simulink model "Project5_openloop"  (R2014b)
settings: Solver=ode5  StartTime=0.0  StopTime=10  FixedStep=0.01  RelTol=1e-3
settings Model: Creator=axk7578  LastModifiedBy=axk7578

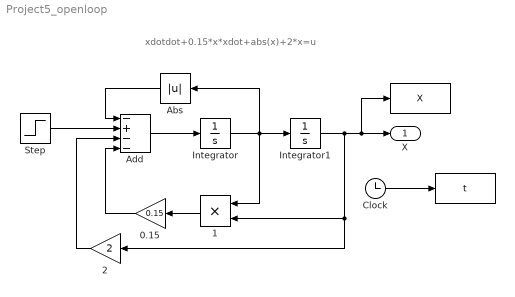
== system Project5_openloop ==
  note: xdotdot+0.15*x*xdot+abs(x)+2*x=u
  " " : ToWorkspace  VariableName=t  SampleTime=-1
  " " : ToWorkspace  VariableName=X  SampleTime=-1
  " 1" : Product
  0.15 : Gain  Gain=0.15
  2 : Gain  Gain=2
  Abs : Abs
  Add : Sum  Inputs=-+--
  Clock : Clock
  Integrator : Integrator
  Integrator1 : Integrator
  Step : Step  Time=0  SampleTime=0
  X : Outport
  wires:
  Clock/1 -> " "/1
  Integrator/1 -> Abs/1, " 1"/1, Integrator1/1
  Integrator1/1 -> 2/1, " 1"/2, " "/1, X/1
  Add/1 -> Integrator/1
  " 1"/1 -> 0.15/1
  0.15/1 -> Add/4
  Step/1 -> Add/2
  Abs/1 -> Add/1
  2/1 -> Add/3
